simulink model "simulation_TF"  (R2025b)
settings: Solver=VariableStepAuto  StartTime=0.0  StopTime=20  RelTol=1e-3
libraries: simulink x2
settings Model: Creator=David  LastModifiedBy=David

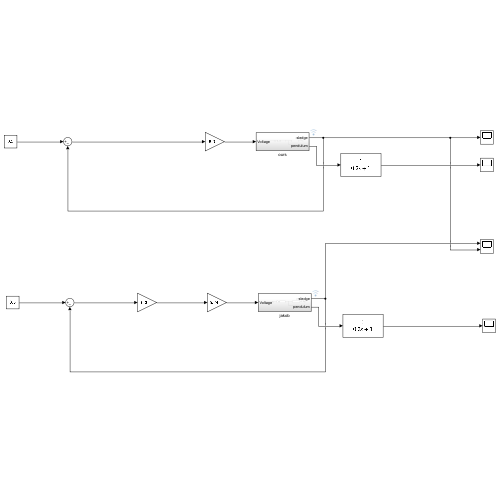
[thumbnail: Simulink's stored preview of the top-level diagram]
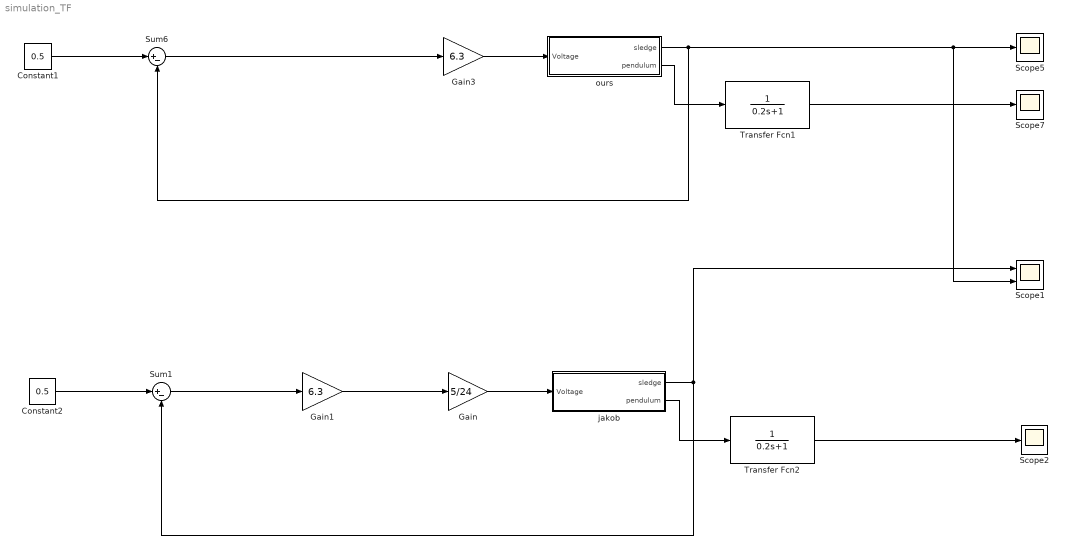
== system simulation_TF ==
  Constant1 : Constant  Value=0.5
  Constant2 : Constant  Value=0.5
  Gain : Gain  Gain=5/24
  Gain1 : Gain  Gain=6.3
  Gain3 : Gain  Gain=6.3
  Scope1 : Scope  NumInputPorts=2
      settings: ActiveDisplayYMinimum=-0.062409174224813728  ActiveDisplayYMaximum=0.56168256802332373
  Scope2 : Scope
      settings: ActiveDisplayYMinimum=-0.079352765901140043  ActiveDisplayYMaximum=0.10008467304526525
  Scope5 : Scope
      settings: ActiveDisplayYMinimum=-0.062409174224813728  ActiveDisplayYMaximum=0.56168256802332373  DataLoggingVariableName=ScopeData5
  Scope7 : Scope
      settings: ActiveDisplayYMinimum=-0.079352765901140043  ActiveDisplayYMaximum=0.10008467304526525  DataLoggingVariableName=ScopeData7
  Sum1 : Sum  Inputs=|+-
  Sum6 : Sum  Inputs=|+-
  Transfer Fcn1 : TransferFcn  Denominator=[0.2 1]
  Transfer Fcn2 : TransferFcn  Denominator=[0.2 1]
  jakob : Subsystem
  ours : Subsystem
  wires:
  ours/1(sledge) -> Scope1/2, Scope5/1, Sum6/2
  ours/2(pendulum) -> Transfer Fcn1/1
  Gain3/1 -> ours/1(Voltage)
  Constant1/1 -> Sum6/1
  Transfer Fcn1/1 -> Scope7/1
  Sum6/1 -> Gain3/1
  Sum1/1 -> Gain1/1
  Transfer Fcn2/1 -> Scope2/1
  Constant2/1 -> Sum1/1
  Gain1/1 -> Gain/1
  jakob/2(pendulum) -> Transfer Fcn2/1
  jakob/1(sledge) -> Sum1/2, Scope1/1
  Gain/1 -> jakob/1(Voltage)

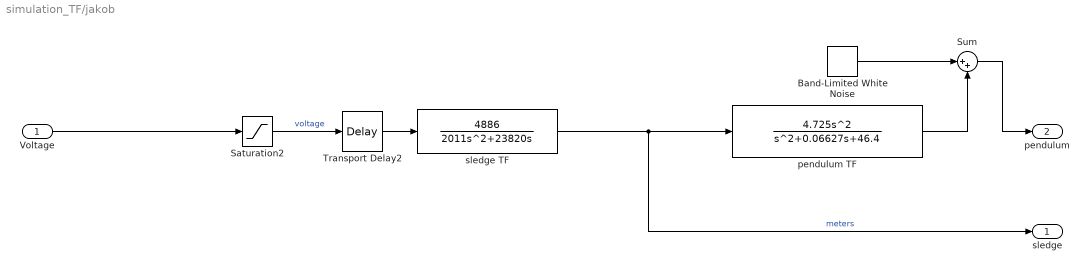
== system simulation_TF/jakob ==
  Voltage : Inport
  Band-Limited White Noise : simulink/Sources/Band-Limited White Noise  Cov=[4.9008e-09]  Ts=0.01  seed=[23341]
  Saturation2 : Saturate  UpperLimit=12  LowerLimit=-12
  Sum : Sum  Inputs=|++
  Transport Delay2 : TransportDelay  DelayTime=0.01
  pendulum TF : TransferFcn  Numerator=[4.725 0 0]  Denominator=[1 0.06627 46.4]
  sledge TF : TransferFcn  Numerator=4886  Denominator=[2011 23820 0]
  sledge : Outport
  pendulum : Outport  Port=2
  wires:
  Transport Delay2/1 -> sledge TF/1
  Voltage/1 -> Saturation2/1
  Sum/1 -> pendulum/1
  Band-Limited White Noise/1 -> Sum/1
  pendulum TF/1 -> Sum/2
  sledge TF/1 -> sledge/1, pendulum TF/1  "meters"
  Saturation2/1 -> Transport Delay2/1  "voltage"

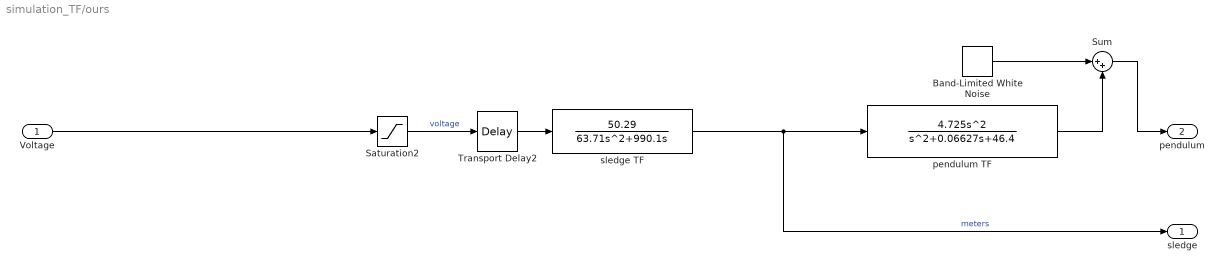
== system simulation_TF/ours ==
  Voltage : Inport
  Band-Limited White Noise : simulink/Sources/Band-Limited White Noise  Cov=[4.9008e-09]  Ts=0.01  seed=[23341]
  Saturation2 : Saturate  UpperLimit=12  LowerLimit=-12
  Sum : Sum  Inputs=|++
  Transport Delay2 : TransportDelay  DelayTime=0.01
  pendulum TF : TransferFcn  Numerator=[4.725 0 0]  Denominator=[1 0.06627 46.4]
  sledge TF : TransferFcn  Numerator=50.29  Denominator="[63.71  990.1 0]"
  sledge : Outport
  pendulum : Outport  Port=2
  wires:
  Saturation2/1 -> Transport Delay2/1  "voltage"
  sledge TF/1 -> pendulum TF/1, sledge/1  "meters"
  pendulum TF/1 -> Sum/2
  Band-Limited White Noise/1 -> Sum/1
  Sum/1 -> pendulum/1
  Voltage/1 -> Saturation2/1
  Transport Delay2/1 -> sledge TF/1
